simulink model "controller_arduino"  (R2021b)
settings: Solver=FixedStepAuto  StartTime=0.0  StopTime=10.0  FixedStep=1/10  RelTol=1e-3  EnableMultiTasking=on
libraries: arduinolib x6
settings Model: ExtModeTrigDuration=2  Creator=DAUIN-Win10  LastModifiedBy=DAUIN-Win10
settings OptimizationCC: EnhancedBackFolding=on  PassReuseOutputArgsAs=Individual arguments  ZeroExternalMemoryAtStartup=off  ZeroInternalMemoryAtStartup=off  MaxStackSize=64  OptimizeBlockOrder=speed  DifferentSizesBufferReuse=on  OptimizationCustomize=off  EfficientTunableParamExpr=on
settings DebuggingCC: ParameterTunabilityLossMsg=error
settings HardwareCC: ProdBitPerInt=16  ProdBitPerPointer=16  ProdBitPerSizeT=16  ProdBitPerPtrDiffT=16  ProdLargestAtomicFloat=None  ProdWordSize=8  ProdHWDeviceType=Atmel->AVR
settings SFSimCC: MATLABDynamicMemAlloc=off
settings RTWCC: Description=Embedded Coder  SystemTargetFile=ert.tlc  HardwareBoard=Arduino Uno  TemplateMakefile=ert_default_tmf  Toolchain=Arduino AVR  BuildConfiguration=Faster Runs
settings CodeAppCC: ForceParamTrailComments=on  IgnoreCustomStorageClasses=off  OperatorAnnotations=on  SimulinkDataObjDesc=on  SFDataObjDesc=on  InsertBlockDesc=on
settings ERTTargetCC: SupportContinuousTime=on  SupportVariableSizeSignals=on  ExtModeTransport=3  ExtModeStaticAlloc=on  ExtModeStaticAllocSize=250  ExtModeMexFile=ext_xcp  ExtModeIntrfLevel=Level2 - Open

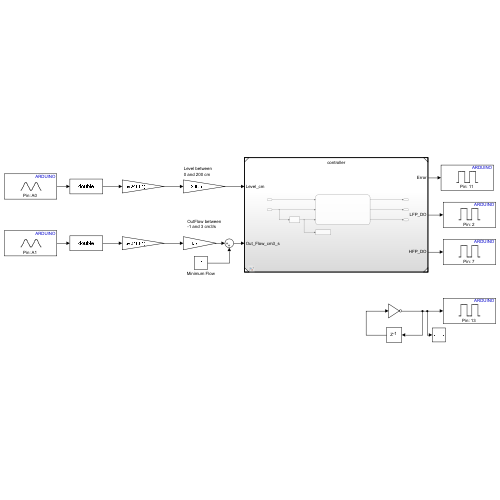
[thumbnail: Simulink's stored preview of the top-level diagram]
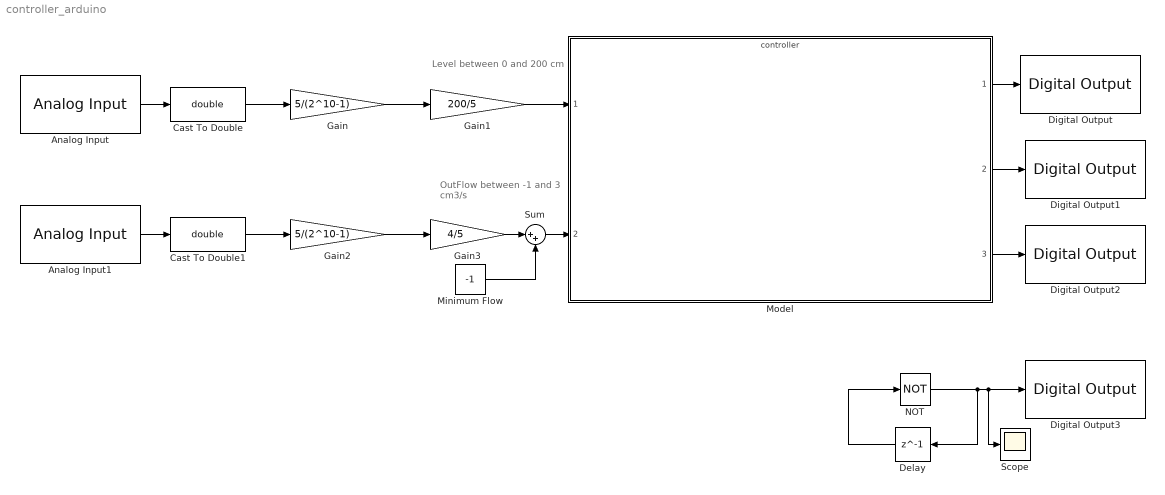
== system controller_arduino ==
  note: Level between
      | 0 and 200 cm
  note: OutFlow between
      | -1 and 3 cm3/s
  Analog Input : arduinolib/Analog Input  pinNumber=0  ReadResultsOnly=off  ConversionTriggerSource=Software  ExternalTriggerType=uint32( 0 )  OutputDataType=uint16  EnableConversionCompleteNotify=off  EnableOuputStatus=off  SampleTime=-1  blockPlatform=arduino
  Analog Input1 : arduinolib/Analog Input  pinNumber=1  ReadResultsOnly=off  ConversionTriggerSource=Software  ExternalTriggerType=uint32( 0 )  OutputDataType=uint16  EnableConversionCompleteNotify=off  EnableOuputStatus=off  SampleTime=-1  blockPlatform=arduino
  Cast To Double : DataTypeConversion  OutDataTypeStr=double
  Cast To Double1 : DataTypeConversion  OutDataTypeStr=double
  Delay : Delay  DelayLength=1  SampleTime=0.5
  Digital Output : arduinolib/Digital Output  pinNumber=11  Direction=output  blockPlatform=arduino
  Digital Output1 : arduinolib/Digital Output  pinNumber=2  Direction=output  blockPlatform=arduino
  Digital Output2 : arduinolib/Digital Output  pinNumber=7  Direction=output  blockPlatform=arduino
  Digital Output3 : arduinolib/Digital Output  pinNumber=13  Direction=output  blockPlatform=arduino
  Gain : Gain  Gain=5/(2^10-1)
  Gain1 : Gain  Gain=200/5
  Gain2 : Gain  Gain=5/(2^10-1)
  Gain3 : Gain  Gain=4/5
  Minimum Flow : Constant  Value=-1
  Model : ModelReference  ModelNameDialog=controller  SimulationMode=Normal  ModelReferenceVersion=1.10
  NOT : Logic  Operator=NOT  IconShape=distinctive  AllPortsSameDT=off  OutDataTypeStr=boolean
  Scope : Scope
  Sum : Sum  Inputs=|++
  wires:
  Model/1 -> Digital Output/1
  Model/2 -> Digital Output1/1
  Model/3 -> Digital Output2/1
  Analog Input/1 -> Cast To Double/1
  Cast To Double/1 -> Gain/1
  Gain/1 -> Gain1/1
  Gain1/1 -> Model/1
  Cast To Double1/1 -> Gain2/1
  Analog Input1/1 -> Cast To Double1/1
  Gain2/1 -> Gain3/1
  Gain3/1 -> Sum/1
  Sum/1 -> Model/2
  Minimum Flow/1 -> Sum/2
  NOT/1 -> Delay/1, Scope/1, Digital Output3/1
  Delay/1 -> NOT/1
